simulink model "Step_Response_2_2"  (Simulink 7.7)
settings: Solver=ode45  StartTime=0.0  StopTime=10  RelTol=1e-3
libraries: simulink x1
settings Model: Creator=Kaustubh C Shivdikar  LastModifiedBy=Kaustubh C Shivdikar

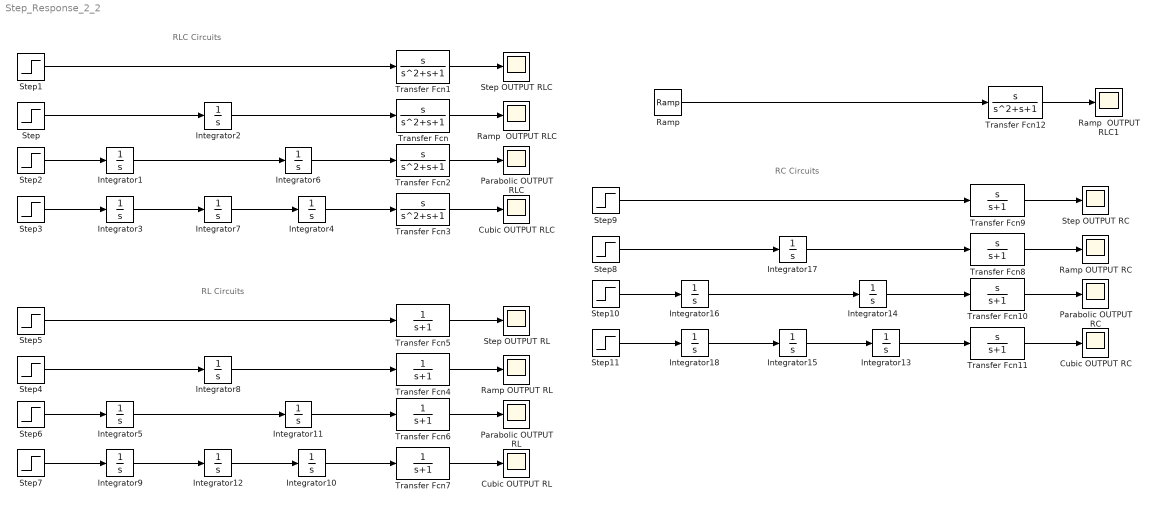
== system Step_Response_2_2 ==
  note: RLC Circuits
  note: RL Circuits
  note: RC Circuits
  Cubic OUTPUT RC : Scope
      settings: SaveName=ScopeData9
  Cubic OUTPUT RL : Scope
      settings: SaveName=ScopeData7
  Cubic OUTPUT RLC : Scope
      settings: SaveName=ScopeData3
  Integrator{1..18} (18 alike) : Integrator
  Parabolic OUTPUT RC : Scope
      settings: SaveName=ScopeData8
  Parabolic OUTPUT RL : Scope
      settings: SaveName=ScopeData6
  Parabolic OUTPUT RLC : Scope
      settings: SaveName=ScopeData2
  Ramp : simulink/Sources/Ramp  SystemSampleTime=-1  slope=1  start=0  X0=0
  Ramp  OUTPUT RLC : Scope
  Ramp  OUTPUT RLC1 : Scope
      settings: SaveName=ScopeData12
  Ramp OUTPUT RC : Scope
      settings: SaveName=ScopeData10
  Ramp OUTPUT RL : Scope
      settings: SaveName=ScopeData4
  Step{,1..6,8..11} (11 alike) : Step  Time=0  SampleTime=0
  Step OUTPUT RC : Scope
      settings: SaveName=ScopeData11
  Step OUTPUT RL : Scope
      settings: SaveName=ScopeData5
  Step OUTPUT RLC : Scope
  Step7 : Step  Time=0  SampleTime=0  VectorParams1D=off
  Transfer Fcn{,1..3,12} (5 alike) : TransferFcn  Numerator=[1 0]  Denominator=[1 1 1]
  Transfer Fcn{8..11} (4 alike) : TransferFcn  Numerator=[1 0]  Denominator=[1 1]
  Transfer Fcn{4..7} (4 alike) : TransferFcn  Denominator=[1 1]
  wires:
  Transfer Fcn/1 -> Ramp  OUTPUT RLC/1
  Step1/1 -> Transfer Fcn1/1
  Transfer Fcn1/1 -> Step OUTPUT RLC/1
  Transfer Fcn2/1 -> Parabolic OUTPUT RLC/1
  Step/1 -> Integrator2/1
  Integrator2/1 -> Transfer Fcn/1
  Step2/1 -> Integrator1/1
  Integrator1/1 -> Integrator6/1
  Integrator6/1 -> Transfer Fcn2/1
  Transfer Fcn3/1 -> Cubic OUTPUT RLC/1
  Step3/1 -> Integrator3/1
  Integrator3/1 -> Integrator7/1
  Integrator7/1 -> Integrator4/1
  Integrator4/1 -> Transfer Fcn3/1
  Transfer Fcn4/1 -> Ramp OUTPUT RL/1
  Step5/1 -> Transfer Fcn5/1
  Transfer Fcn5/1 -> Step OUTPUT RL/1
  Transfer Fcn6/1 -> Parabolic OUTPUT RL/1
  Step4/1 -> Integrator8/1
  Integrator8/1 -> Transfer Fcn4/1
  Step6/1 -> Integrator5/1
  Integrator5/1 -> Integrator11/1
  Integrator11/1 -> Transfer Fcn6/1
  Transfer Fcn7/1 -> Cubic OUTPUT RL/1
  Step7/1 -> Integrator9/1
  Integrator9/1 -> Integrator12/1
  Integrator12/1 -> Integrator10/1
  Integrator10/1 -> Transfer Fcn7/1
  Transfer Fcn8/1 -> Ramp OUTPUT RC/1
  Step9/1 -> Transfer Fcn9/1
  Transfer Fcn9/1 -> Step OUTPUT RC/1
  Transfer Fcn10/1 -> Parabolic OUTPUT RC/1
  Step8/1 -> Integrator17/1
  Integrator17/1 -> Transfer Fcn8/1
  Step10/1 -> Integrator16/1
  Integrator16/1 -> Integrator14/1
  Integrator14/1 -> Transfer Fcn10/1
  Transfer Fcn11/1 -> Cubic OUTPUT RC/1
  Step11/1 -> Integrator18/1
  Integrator18/1 -> Integrator15/1
  Integrator15/1 -> Integrator13/1
  Integrator13/1 -> Transfer Fcn11/1
  Transfer Fcn12/1 -> Ramp  OUTPUT RLC1/1
  Ramp/1 -> Transfer Fcn12/1
